simulink model "power_3pfault_parametertest"  (R2017b)
settings: Solver=FixedStepDiscrete  StartTime=0.0  StopTime=0.2  FixedStep=Ts  RelTol=1e-4  EnableMultiTasking=on
PreLoadFcn:
  | Ts=50e-6;
InitFcn:
  | Ts=50e-6;
undefined symbols (not defined in the file or in its folder): D1, Delta
libraries: powerlib x23
Description:
  | Copyright 2008-2017 The MathWorks, Inc.
settings Model: ExtModeTrigMode=oneshot  ExtModeArmWhenConnect=off  ExtModeAutoUpdateStatusClock=off  Creator=MathWorks  LastModifiedBy=estheim
settings DataIOCC: SaveFormat=Array  SignalLoggingSaveFormat=ModelDataLogs  SignalLoggingName=sigsOut
settings OptimizationCC: BlockReduction=off  BooleanDataType=off  ExpressionDepthLimit=2147483647  InitFltsAndDblsToZero=on  EfficientMapNaN2IntZero=off  LifeSpan=inf
settings DebuggingCC: UnderspecifiedInitializationDetection=Classic  MergeDetectMultiDrivingBlocksExec=none  CheckExecutionContextPreStartOutputMsg=on  CheckExecutionContextRuntimeOutputMsg=on  SignalResolutionControl=TryResolveAllWithWarning  MultiTaskDSMMsg=warning  MultiTaskCondExecSysMsg=none  FcnCallInpInsideContextMsg=warning  UnconnectedInputMsg=none  UnconnectedOutputMsg=none  StateNameClashWarn=warning  SFUnexpectedBacktrackingDiag=warning  SFNoUnconditionalDefaultTransitionDiag=warning  SFExecutionAtInitializationDiag=none
settings HardwareCC: ProdBitPerPointer=32  ProdBitPerSizeT=32  ProdBitPerPtrDiffT=32  ProdLargestAtomicFloat=None  ProdIntDivRoundTo=Undefined  ProdEndianess=Unspecified  ProdWordSize=32  ProdHWDeviceType=Specified  TargetUnknown=on
settings ModelReferenceCC: PropagateSignalLabelsOutOfModel=off
settings CodeAppCC: StateflowObjectComments=on
settings GRTTargetCC: TargetLangStandard=C89/C90 (ANSI)  GeneratePreprocessorConditionals=Disable all  CombineOutputUpdateFcns=off  GRTInterface=on
settings ConfigComp: CovMetricSettings=dw  CovHtmlReporting=on  CovSaveCumulativeToWorkspaceVar=on  CovSaveSingleToWorkspaceVar=on  CovExternalEMLEnable=off  CovSFcnEnable=off
settings SimscapeCC: SimscapeNormalizeSystem=off

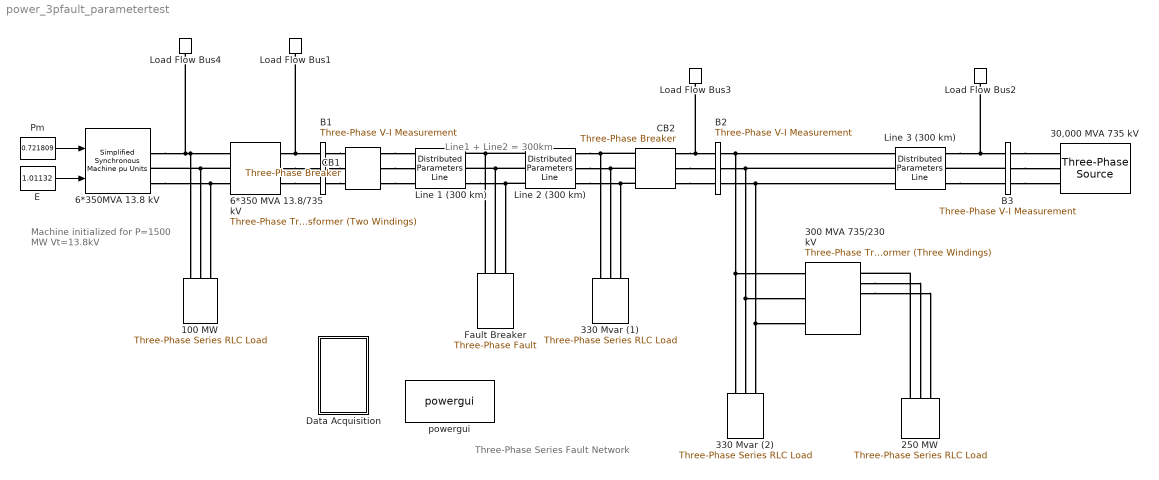
== system power_3pfault_parametertest ==
  note: Line1 + Line2 = 300km
  note: Machine initialized for
      |  P=1500 MW
      |  Vt=13.8kV
  note: Three-Phase Series Fault Network
  100 MW : powerlib/Elements/Three-Phase Series RLC Load  LConnTagsString=A|B|C  Configuration=Y (grounded)  NominalVoltage=13.8e3  Vabc=[1e3 1e3 1e3]  Vabcp=[1e3 1e3 1e3]  NominalFrequency=60  UnbalancedPower=off  ActivePower=100000000  InductivePower=0  CapacitivePower=0  Pabc=[10e3 9e3 11e3]  QLabc=[100 90 110]  QCabc=[100 90 110]  Pabcp=[10e3 9e3 11e3]  QLabcp=[100 90 110]  QCabcp=[100 90 110]  Measurements=None  LoadType=constant Z
  250 MW : powerlib/Elements/Three-Phase Series RLC Load  LConnTagsString=A|B|C  Configuration=Y (grounded)  NominalVoltage=230e3  Vabc=[1e3 1e3 1e3]  Vabcp=[1e3 1e3 1e3]  NominalFrequency=60  UnbalancedPower=off  ActivePower=250000000  InductivePower=0  CapacitivePower=0  Pabc=[10e3 9e3 11e3]  QLabc=[100 90 110]  QCabc=[100 90 110]  Pabcp=[10e3 9e3 11e3]  QLabcp=[100 90 110]  QCabcp=[100 90 110]  Measurements=None  LoadType=constant Z
  30,000 MVA 735 kV : powerlib/Electrical Sources/Three-Phase Source  InternalConnection=Yg  VoltagePhases=off  Voltage=(735000)*0.98865  PhaseAngle=-2.0892  Voltage_phases=[25e3 25e3 25e3]/sqrt(3)  PhaseAngles_phases=[0 -120 +120]  Frequency=60  NonIdealSource=on  SpecifyImpedance=on  Resistance=735^2/30000/10  Inductance=735^2/30000/377  ShortCircuitLevel=30000e6  BaseVoltage=735e3  XRratio=10  BusType=swing  Pref=0  Qref=0  Prefabc=[10e3, 10e3, 10e3]  Qrefabc=[0, 0, 0]  Qmin=-Inf  Qmax=Inf
  300 MVA 735/230 kV : powerlib/Elements/Three-Phase Transformer (Three Windings)  Winding1Connection=Yg  Winding2Connection=Yg  Winding3Connection=Delta (D1)  CoreType=Three single-phase transformers  SetSaturation=on  Hysteresis=off  DataFile='hysteresis'  SetInitialFlux=off  Measurements=None  UNITS=pu  NominalPower=[ 300e6 , 60 ]  Winding1=[ 735e3 , 0.002 , 0.15 ]  Winding2=[ 230e3 , 0.002 , 0 ]  Winding3=[ 25e3 , 0.05 , 0.20 ]  Rm=500  Lm=1000  L0=0.5  Saturation="[  0,0  ;  0.0012,1.2  ;  1.0,1.45 ]"  InitialFluxes=[-1.0077512712612 0.407399313381507 0.600351957879682]  MoreParameters=on  BreakLoop=on  DataType=off  TransfoNumber=0
      settings: AttributesFormatString=\n  SourceProductName=Simscape Power Systems  SourceProductBaseCode=PS
  330 Mvar (1) : powerlib/Elements/Three-Phase Series RLC Load  LConnTagsString=A|B|C  Configuration=Y (grounded)  NominalVoltage=735e3  Vabc=[1e3 1e3 1e3]  Vabcp=[1e3 1e3 1e3]  NominalFrequency=60  UnbalancedPower=off  ActivePower=1320000  InductivePower=330e6  CapacitivePower=0  Pabc=[10e3 9e3 11e3]  QLabc=[100 90 110]  QCabc=[100 90 110]  Pabcp=[10e3 9e3 11e3]  QLabcp=[100 90 110]  QCabcp=[100 90 110]  Measurements=None  LoadType=constant Z
  "330 Mvar (2) " : powerlib/Elements/Three-Phase Series RLC Load  LConnTagsString=A|B|C  Configuration=Y (grounded)  NominalVoltage=735e3  Vabc=[1e3 1e3 1e3]  Vabcp=[1e3 1e3 1e3]  NominalFrequency=60  UnbalancedPower=off  ActivePower=1320000  InductivePower=330e6  CapacitivePower=0  Pabc=[10e3 9e3 11e3]  QLabc=[100 90 110]  QCabc=[100 90 110]  Pabcp=[10e3 9e3 11e3]  QLabcp=[100 90 110]  QCabcp=[100 90 110]  Measurements=None  LoadType=constant Z
  6*350 MVA 13.8/735 kV : powerlib/Elements/Three-Phase Transformer (Two Windings)  Winding1Connection=Delta (D1)  Winding2Connection=Yg  CoreType=Three single-phase transformers  SetSaturation=off  Hysteresis=off  DataFile='hysteresis'  SetInitialFlux=off  Measurements=None  UNITS=pu  NominalPower=[ 6*350e6 , 60 ]  Winding1=[ 13.8e3 , 0.002 , 0.08 ]  Winding2=[ 735e3 , 0.002 , 0.08 ]  Rm=500  Lm=500  L0=0.5  Saturation=[ 0,0 ; 0.0024,1.2 ; 1.0,1.52 ]  InitialFluxes=[ 0.8 , -0.8 , 0.7 ]  MoreParameters=off  BreakLoop=off  DataType=off  TransfoNumber=0
  6*350MVA 13.8 kV : powerlib/Machines/Simplified Synchronous Machine pu Units  ConnectionType=3-wire Y  MechanicalLoad=Mechanical power Pm  MeasurementBus=off  NominalParameters="[ 6*350e6 13.8e3  60 ]"  Mechanical=[ inf,0,2 ]  InternalRL="[ 0.22/15  0.22 ]"  InitialConditions=[0 1.43122 0.716215 0.716215 0.716215 -3.34575 -123.346 116.654 ]  Units=0  LoadFlowParameters=[1,0,0,0,0]  TsPowergui=0  TsBlock=-1  BusType=PV  Pref=1500000000  Qref=0  Qmin=-Inf  Qmax=Inf  PLF=0  QLF=0
      settings: AttributesFormatString=\n  SourceProductName=Simscape Power Systems  SourceProductBaseCode=PS
  B1 : powerlib/Measurements/Three-Phase V-I Measurement  VoltageMeasurement=phase-to-ground  SetLabelV=on  LabelV=Vabc_B1  Vpu=on  VpuLL=off  CurrentMeasurement=yes  SetLabelI=on  LabelI=Iabc_B1  Ipu=on  Pbase=100e6  Vbase=735e3  OutputType=Complex  PhasorSimulation=off  PSBequivalent=0
  B2 : powerlib/Measurements/Three-Phase V-I Measurement  VoltageMeasurement=phase-to-ground  SetLabelV=on  LabelV=Vabc_B2  Vpu=on  VpuLL=off  CurrentMeasurement=yes  SetLabelI=on  LabelI=Iabc_B2  Ipu=on  Pbase=100e6  Vbase=735e3  OutputType=Complex  PhasorSimulation=off  PSBequivalent=0
  B3 : powerlib/Measurements/Three-Phase V-I Measurement  VoltageMeasurement=no  SetLabelV=on  LabelV=Vabc_B3  Vpu=on  VpuLL=off  CurrentMeasurement=no  SetLabelI=on  LabelI=Iabc_B3  Ipu=on  Pbase=100e6  Vbase=735e3  OutputType=Complex  PhasorSimulation=off  PSBequivalent=0
  CB1 : powerlib/Elements/Three-Phase Breaker  InitialState=closed  SwitchA=on  SwitchB=on  SwitchC=on  SwitchTimes="[5/60  ]"  External=off  BreakerResistance=0.001  SnubberResistance=1e5  SnubberCapacitance=inf  Measurements=None
      settings: AttributesFormatString=\n
  CB2 : powerlib/Elements/Three-Phase Breaker  InitialState=closed  SwitchA=on  SwitchB=on  SwitchC=on  SwitchTimes="[5/60  ]"  External=off  BreakerResistance=0.001  SnubberResistance=1e5  SnubberCapacitance=inf  Measurements=None
      settings: AttributesFormatString=\n
  Data Acquisition : Subsystem  mask(Data Acquisition){}
      mask Display: disp('Scopes')
  E : Constant  Value=1.01132
  Fault Breaker : powerlib/Elements/Three-Phase Fault  InitialStates=0  FaultA=off  FaultB=on  FaultC=off  GroundFault=on  SwitchTimes=faultinception2  External=off  SwitchStatus=NaN  FaultResistance=faultres  GroundResistance=1  SnubberResistance=inf  SnubberCapacitance=inf  Measurements=Fault voltages and currents
  Line 1 (300 km) : powerlib/Elements/Distributed Parameters Line  Phases=3  Frequency=60  Resistance=[0.01273 0.3864]  Inductance="[0.9337e-3  4.1264e-3]"  Capacitance=[12.74e-9 7.751e-9]  Length=line1  x1=[-0.0003 -3.78759842950766e-08 628975.403312343 -495883.769880965;-0.00025 -3.75285463548764e-08 638210.318952053 -483940.521945147;-0.0002 -3.71677747008528e-08 647218.481504353 -471825.332246222;-0.00015 -3.67937975134568e-08 655996.690411981 -459542.505253402;-0.0001 -3.64067476650022e-08 664541.826819112 -447096.404996632;-5e-05 -3.60067626724573e-08 672850.854679469 -434491.453516068]  x2=[-0.0003 -3.45807686958301e-08 605295.232742086 -519409.81725687;-0.00025 -3.4265507824739e-08 614977.783461343 -507908.720868203;-0.0002 -3.39380725818771e-08 624441.835502426 -496227.166929478;-0.00015 -3.3598579303427e-08 633684.026332709 -484369.305841187;-0.0001 -3.32471486097339e-08 642701.072245797 -472339.350644913;-5e-05 -3.28839053624501e-08 651489.769528212 -460141.575526454]  x3=[-0.0003 -2.61251237348243e-11 876.888880838957 -609.09527519692;-0.00025 -2.50551766038549e-11 888.21347189918 -592.459310580762;-0.0002 -2.39763274879413e-11 899.22248494217 -575.612847992619;-0.00015 -2.28889596970374e-11 909.912008518013 -558.561872900433;-0.0001 -2.17934595677416e-11 920.278244689884 -541.312443434463;-5e-05 -2.06902163260335e-11 930.31751038343 -523.870688234865]  x4=[-0.0003 -7.92696517991683e-11 3552.49798963012 -3282.73159030779;-0.00025 -7.95960668313405e-11 3613.74152071813 -3215.18949934517;-0.0002 -7.98942017599735e-11 3673.7011066511 -3146.50506686293;-0.00015 -8.0163950659147e-11 3732.35544407363 -3076.70269611289;-0.0001 -8.04052176883613e-11 3789.68369337894 -3005.80718754501;-5e-05 -8.06179171265899e-11 3845.66548611301 -2933.8437299959]  x5=0.000282770783497871  V1=ones(3,3)  V2=ones(3,3)  I1=ones(3,3)  I2=ones(3,3)  nHarmo=1  Measurements=None
      settings: AttributesFormatString=\n  SourceProductName=Simscape Power Systems
  Line 2 (300 km) : powerlib/Elements/Distributed Parameters Line  Phases=3  Frequency=60  Resistance=[0.01273 0.3864]  Inductance="[0.9337e-3  4.1264e-3]"  Capacitance=[12.74e-9 7.751e-9]  Length=line2  x1=[-0.00145 -3.82709877736309e-08 0 0;-0.0014 -3.82574787054797e-08 0 0;-0.00135 -3.8230376937312e-08 0 0;-0.0013 -3.81896920982569e-08 0 0;-0.00125 -3.8135438643444e-08 0 0;-0.0012 -3.80676358488675e-08 0 0;-0.00115 -3.79863078045374e-08 0 0;-0.0011 -3.78914834059206e-08 0 0;-0.00105 -3.77831963436745e-08 0 0;-0.001 -3.76614850916767e-08 0 0;-0.00095 -3.75263928933554e-08 0 0;-0.0009 -3.73779677463254e-08 473387.852694452 -641928.29724098;-0.00085 -3.72162623853347e-08 485403.128607504 -632891.679417048;-0.0008 -3.70413342635282e-08 497245.943100267 -623630.198193008;-0.00075 -3.68532455320345e-08 508912.088477141 -614147.144129039;-0.0007 -3.66520630178844e-08 520397.419812224 -604445.886509095;-0.00065 -3.64378582002671e-08 531697.856421981 -594529.872143814;-0.0006 -3.62107071851344e-08 542809.383315095 -584402.624145885;-0.00055 -3.59706906781605e-08 553728.052618967 -574067.740678299;-0.0005 -3.57178939560672e-08 564449.984982385 -563528.893675942;-0.00045 -3.54524068363264e-08 574971.370953834 -552789.82754097;-0.0004 -3.51743236452474e-08 585288.472334977 -541854.357812448;-0.00035 -3.48837431844639e-08 595397.62350882 -530726.369810698;-0.0003 -3.45807686958301e-08 605295.232742086 -519409.81725687;-0.00025 -3.4265507824739e-08 614977.783461343 -507908.720868203;-0.0002 -3.39380725818771e-08 624441.835502426 -496227.166929478;-0.00015 -3.3598579303427e-08 633684.026332709 -484369.305841187;-0.0001 -3.32471486097339e-08 642701.072245797 -472339.350644913;-5e-05 -3.28839053624501e-08 651489.769528212 -460141.575526454]  x2=[-0.00145 -1.47649338361576e-08 0 0;-0.0014 -1.47608425428165e-08 0 0;-0.00135 -1.47515067924054e-08 0 0;-0.0013 -1.4736929901872e-08 0 0;-0.00125 -1.47171170503161e-08 0 0;-0.0012 -1.46920752771496e-08 0 0;-0.00115 -1.46618134795951e-08 0 0;-0.0011 -1.46263424095253e-08 0 0;-0.00105 -1.45856746696424e-08 0 0;-0.001 -1.45398247090008e-08 0 0;-0.00095 -1.44888088178732e-08 0 0;-0.0009 -1.44326451219628e-08 305808.693622115 -687287.971048075;-0.00085 -1.43713535759632e-08 318708.688794987 -681401.883166662;-0.0008 -1.43049559564691e-08 331495.448288299 -675273.696440736;-0.00075 -1.42334758542383e-08 344164.429027289 -668905.58818586;-0.0007 -1.41569386658109e-08 356711.129783425 -662299.820960574;-0.00065 -1.40753715844855e-08 369131.092773671 -655458.74176252;-0.0006 -1.39888035906577e-08 381419.905244316 -648384.781194561;-0.00055 -1.38972654415234e-08 393573.201038804 -641080.452601205;-0.0005 -1.38007896601512e-08 405586.662149007 -633548.35117562;-0.00045 -1.36994105239269e-08 417456.020249398 -625791.153037578;-0.0004 -1.35931640523748e-08 429177.058213561 -617811.614282639;-0.00035 -1.34820879943603e-08 440745.611612517 -609612.570002929;-0.0003 -1.3366221814678e-08 452157.57019433 -601196.933279839;-0.00025 -1.32456066800298e-08 463408.879344454 -592567.694149025;-0.0002 -1.31202854443986e-08 474495.541526323 -583727.918538061;-0.00015 -1.29903026338229e-08 485413.617701655 -574680.747177129;-0.0001 -1.28557044305762e-08 496159.228729971 -565429.394483136;-5e-05 -1.27165386567593e-08 506728.55674684 -555977.147417641]  x3=[-0.00145 -3.38199281059364e-11 0 0;-0.0014 -3.30171295486336e-11 0 0;-0.00135 -3.22026001624171e-11 0 0;-0.0013 -3.13766293456994e-11 0 0;-0.00125 -3.05395105619787e-11 0 0;-0.0012 -2.96915412355729e-11 0 0;-0.00115 -2.88330226459457e-11 0 0;-0.0011 -2.79642598206644e-11 0 0;-0.00105 -2.70855614270239e-11 0 0;-0.001 -2.61972396623794e-11 0 0;-0.00095 -2.52996101432242e-11 0 0;-0.0009 -2.43929917930521e-11 757.656727728583 -729.222631766939;-0.00085 -2.34777067290461e-11 771.266751177753 -714.812683047661;-0.0008 -2.25540801476311e-11 784.602747222709 -700.148764785762;-0.00075 -2.16224402089336e-11 797.659977647554 -685.236087001576;-0.0007 -2.06831179201877e-11 810.433803280494 -670.07994809851;-0.00065 -1.97364470181298e-11 822.919685642104 -654.68573298055;-0.0006 -1.87827638504238e-11 835.113188557834 -639.058911139025;-0.00055 -1.78224072561581e-11 847.00997973416 -623.205034709326;-0.0005 -1.68557184454577e-11 858.605832297825 -607.12973649826;-0.00045 -1.58830408782542e-11 869.896626297627 -590.838727982736;-0.0004 -1.49047201422556e-11 880.878350168221 -574.337797280508;-0.00035 -1.39211038301611e-11 891.547102155406 -557.632807093684;-0.0003 -1.29325414161627e-11 901.899091702403 -540.729692625733;-0.00025 -1.19393841317789e-11 911.930640796616 -523.634459472741;-0.0002 -1.0941984841064e-11 921.63818527642 -506.353181489645;-0.00015 -9.94069791523649e-12 931.018276097484 -488.891998632227;-0.0001 -8.93587910677354e-12 940.067580558204 -471.257114775611;-5e-05 -7.92788542301321e-12 948.782883483794 -453.454795510062]  x4=[-0.00145 -3.20986509931294e-11 0 0;-0.0014 -3.32576226301539e-11 0 0;-0.00135 -3.4404777992218e-11 0 0;-0.0013 -3.55397095004839e-11 0 0;-0.00125 -3.66620139191907e-11 0 0;-0.0012 -3.77712924989226e-11 0 0;-0.00115 -3.88671511182821e-11 0 0;-0.0011 -3.99492004239198e-11 0 0;-0.00105 -4.10170559688696e-11 0 0;-0.001 -4.20703383491414e-11 0 0;-0.00095 -4.31086733385205e-11 0 0;-0.0009 -4.41316920215295e-11 1294.72060349585 -4606.45046471645;-0.00085 -4.51390309245015e-11 1381.31528161887 -4581.22864876283;-0.0008 -4.61303321447208e-11 1467.41918499962 -4554.37914408437;-0.00075 -4.71052434775842e-11 1553.00172133124 -4525.91149018223;-0.0007 -4.80634185417371e-11 1638.03248354606 -4495.8358014783;-0.00065 -4.90045169021418e-11 1722.48126061917 -4464.16276372154;-0.0006 -4.9928204191032e-11 1806.31804830218 -4430.90363019148;-0.00055 -5.08341522267121e-11 1889.51305978362 -4396.07021769988;-0.0005 -5.17220391301589e-11 1972.03673627207 -4359.67490239234;-0.00045 -5.25915494393834e-11 2053.85975749819 -4321.73061535108;-0.0004 -5.34423742215129e-11 2134.95305213218 -4282.25083800063;-0.00035 -5.42742111825536e-11 2215.28780811258 -4241.24959731787;-0.0003 -5.50867647747943e-11 2294.8354828831 -4198.74146084839;-0.00025 -5.58797463018126e-11 2373.56781353369 -4154.74153153068;-0.0002 -5.66528740210479e-11 2451.45682684215 -4109.26544233011;-0.00015 -5.74058732439029e-11 2528.47484921294 -4062.32935068463;-0.0001 -5.81384764333391e-11 2604.59451650943 -4013.94993276412;-5e-05 -5.88504232989318e-11 2679.78878377629 -3964.14437754538]  x5=0.00141385391748936  V1=ones(3,3)  V2=ones(3,3)  I1=ones(3,3)  I2=ones(3,3)  nHarmo=1  Measurements=None
      settings: AttributesFormatString=\n  SourceProductName=Simscape Power Systems
  Line 3 (300 km) : powerlib/Elements/Distributed Parameters Line  Phases=3  Frequency=60  Resistance=[0.01273 0.3864]  Inductance="[0.9337e-3  4.1264e-3]"  Capacitance=[12.74e-9 7.751e-9]  Length=300  x1=[-0.0017 -1.45723124159187e-08 0 0;-0.00165 -1.45905087920394e-08 0 0;-0.0016 -1.46035212298608e-08 0 0;-0.00155 -1.46113451061256e-08 0 0;-0.0015 -1.46139776410478e-08 0 0;-0.00145 -1.46114178993003e-08 0 0;-0.0014 -1.46036667903472e-08 0 0;-0.00135 -1.45907270681206e-08 0 0;-0.0013 -1.45726033300422e-08 0 0;-0.00125 -1.45493020153897e-08 0 0;-0.0012 -1.45208314030094e-08 0 0;-0.00115 -1.44872016083743e-08 0 0;-0.0011 -1.44484245799902e-08 0 0;-0.00105 -1.44045140951508e-08 266474.832453814 -703471.218755304;-0.001 -1.43554857550421e-08 279686.845489083 -698323.636957029;-0.00095 -1.43013569792e-08 292799.487119911 -692927.944095694;-0.0009 -1.42421469993208e-08 305808.098487165 -687286.057235279;-0.00085 -1.41778768524284e-08 318708.057693168 -681399.980911323;-0.0008 -1.41085693733999e-08 331494.781443838 -675271.806418715;-0.00075 -1.40342491868527e-08 344163.726677113 -668903.711068673;-0.0007 -1.39549426983952e-08 356710.392177076 -662297.957415152;-0.00065 -1.3870678085245e-08 369130.320173217 -655456.892450971;-0.0006 -1.3781485286218e-08 381419.097924258 -648382.946773938;-0.00055 -1.3687395991091e-08 393572.359285978 -641078.633723268;-0.0005 -1.35884436293425e-08 405585.786262486 -633546.548486608;-0.00045 -1.34846633582754e-08 417455.110540379 -625789.367177978;-0.0004 -1.3376092050526e-08 429176.115005258 -617809.845886958;-0.00035 -1.32627682809629e-08 440744.635240049 -609610.81969947;-0.0003 -1.31447323129818e-08 452156.561004597 -601195.201690476;-0.00025 -1.30220260842001e-08 463407.837696017 -592565.981888984;-0.0002 -1.28946931915566e-08 474494.467789275 -583726.226215699;-0.00015 -1.27627788758217e-08 485412.512257488 -574679.075393721;-0.0001 -1.26263300055237e-08 496158.091971445 -565427.743832659;-5e-05 -1.24853950602965e-08 506727.38907784 -555975.518486563]  x2=[-0.0017 -6.87576100037701e-10 0 0;-0.00165 -6.8480237107496e-10 0 0;-0.0016 -6.81785335090544e-10 0 0;-0.00155 -6.78526064022971e-10 0 0;-0.0015 -6.75025715875733e-10 0 0;-0.00145 -6.71285534305859e-10 0 0;-0.0014 -6.67306848182051e-10 0 0;-0.00135 -6.63091071112545e-10 0 0;-0.0013 -6.58639700942858e-10 0 0;-0.00125 -6.53954319223618e-10 0 0;-0.0012 -6.49036590648638e-10 0 0;-0.00115 -6.43888262463464e-10 0 0;-0.0011 -6.38511163844588e-10 0 0;-0.00105 -6.32907205249543e-10 96634.7706415658 -730540.857796646;-0.001 -6.27078377738136e-10 110387.161752313 -728589.667633419;-0.00095 -6.21026752265026e-10 124100.332830112 -726379.613030548;-0.0009 -6.14754478943929e-10 137769.411650574 -723911.479209909;-0.00085 -6.08263786283689e-10 151389.541655082 -721186.143087697;-0.0008 -6.01556980396502e-10 164955.883676299 -718204.572962859;-0.00075 -5.94636444178565e-10 178463.617657503 -714967.828173063;-0.0007 -5.87504636463443e-10 191907.944365128 -711477.05871832;-0.00065 -5.80164091148457e-10 205284.087093914 -707733.504852397;-0.0006 -5.72617416294407e-10 218587.293364039 -703738.496642157;-0.00055 -5.64867293198933e-10 231812.836609661 -699493.453494994;-0.0005 -5.56916475443867e-10 244956.017858239 -694999.883654524;-0.00045 -5.487677879169e-10 258012.16740006 -690259.383664716;-0.0004 -5.40424125807908e-10 270976.646447359 -685273.637802643;-0.00035 -5.3188845358031e-10 283844.848782462 -680044.417480071;-0.0003 -5.23163803917805e-10 296612.202394354 -674573.580614079;-0.00025 -5.14253276646874e-10 309274.171103089 -668863.070966957;-0.0002 -5.05160037635428e-10 321826.256171477 -662914.917455591;-0.00015 -4.95887317667989e-10 334263.99790346 -656731.233430601;-0.0001 -4.86438411297809e-10 346582.977228626 -650314.215925476;-5e-05 -4.76816675676328e-10 358778.817272279 -643666.14487598]  x3=[-0.0017 -1.26865525293809e-11 0 0;-0.00165 -1.22949508567725e-11 0 0;-0.0016 -1.18989808466686e-11 0 0;-0.00155 -1.14987831853282e-11 0 0;-0.0015 -1.10945000610749e-11 0 0;-0.00145 -1.06862751137777e-11 0 0;-0.0014 -1.02742533838165e-11 0 0;-0.00135 -9.85858126055014e-12 0 0;-0.0013 -9.43940643030468e-12 0 0;-0.00125 -9.01687782390138e-12 0 0;-0.0012 -8.59114556374218e-12 0 0;-0.00115 -8.16236091047193e-12 0 0;-0.0011 -7.73067620923624e-12 0 0;-0.00105 -7.29624483555393e-12 146.058519777444 -1136.85216743786;-0.001 -6.85922114082348e-12 167.460346140684 -1133.89743393128;-0.00095 -6.41976039748269e-12 188.802674640324 -1130.53983206561;-0.0009 -5.97801874384112e-12 210.077922448669 -1126.7805547808;-0.00085 -5.5341531286049e-12 231.27853057148 -1122.62093773017;-0.0008 -5.08832125511361e-12 252.396966533639 -1118.06245880587;-0.00075 -4.64068152530903e-12 273.425727055406 -1113.10673761373;-0.0007 -4.19139298345565e-12 294.357340718299 -1107.75553489791;-0.00065 -3.74061525963306e-12 315.184370619652 -1102.01075191526;-0.0006 -3.28850851302011e-12 335.899417014911 -1095.87442975979;-0.00055 -2.83523337499111e-12 356.49511994673 -1089.34874863758;-0.0005 -2.38095089204426e-12 376.964161859926 -1082.43602709203;-0.00045 -1.92582246858266e-12 397.299270201372 -1075.1387211802;-0.0004 -1.47000980956799e-12 417.493220003902 -1067.45942360014;-0.00035 -1.01367486306761e-12 437.538836453309 -1059.40086276971;-0.0003 -5.56979762715121e-13 457.428997437517 -1050.9659018572;-0.00025 -1.0008677010506e-13 477.156636077037 -1042.15753776405;-0.0002 3.56841782857845e-13 496.714743235796 -1032.9789000601;-0.00015 8.13643551634444e-13 516.09637001145 -1023.4332498716;-0.0001 1.27015623673141e-12 535.294630204293 -1013.52397872262;-5e-05 1.72621764136546e-12 554.302702763892 -1003.25460733002]  x4=[-0.0017 -4.82541696893376e-12 0 0;-0.00165 -5.35583900695815e-12 0 0;-0.0016 -5.88435814088582e-12 0 0;-0.00155 -6.41078659038511e-12 0 0;-0.0015 -6.93493731793454e-12 0 0;-0.00145 -7.45662409527644e-12 0 0;-0.0014 -7.97566156958288e-12 0 0;-0.00135 -8.49186532931071e-12 0 0;-0.0013 -9.00505196972204e-12 0 0;-0.00125 -9.51503915804716e-12 0 0;-0.0012 -1.00216456982664e-11 0 0;-0.00115 -1.05246915954883e-11 0 0;-0.0011 -1.10239981199009e-11 0 0;-0.00105 -1.15193878702735e-11 141.875750296584 -4366.85509796771;-0.001 -1.20106848369868e-11 224.159158139472 -4363.40508133909;-0.00095 -1.24977144645678e-11 306.362923300832 -4358.40476766195;-0.0009 -1.29803037137088e-11 388.457839174327 -4351.85593352391;-0.00085 -1.34582811227476e-11 470.414737827251 -4343.76090569457;-0.0008 -1.39314768685867e-11 552.204500363761 -4334.12256029876;-0.00075 -1.43997228270308e-11 633.798067270678 -4322.94432179472;-0.0007 -1.48628526325204e-11 715.166448742199 -4310.23016175735;-0.00065 -1.53207017372409e-11 796.28073497983 -4295.98459746718;-0.0006 -1.57731074695855e-11 877.112106463908 -4280.21269030536;-0.00055 -1.62199090919516e-11 957.631844193032 -4262.92004395542;-0.0005 -1.66609478578504e-11 1037.81133988779 -4244.11280241226;-0.00045 -1.70960670683084e-11 1117.62210615515 -4223.79764779925;-0.0004 -1.7525112127542e-11 1197.03578660988 -4201.98179799408;-0.00035 -1.79479305978845e-11 1276.02416594946 -4178.67300406432;-0.0003 -1.83643722539467e-11 1354.55917997881 -4153.87954751346;-0.00025 -1.87742891359913e-11 1432.61292558141 -4127.61023733856;-0.0002 -1.91775356025019e-11 1510.15767063311 -4099.87440690043;-0.00015 -1.95739683819289e-11 1587.16586385522 -4070.68191060756;-0.0001 -1.99634466235937e-11 1663.61014460339 -4040.04312041489;-5e-05 -2.03458319477314e-11 1739.46335258865 -4007.96892213868]  x5=0.00169662470098723  V1=ones(3,3)  V2=ones(3,3)  I1=ones(3,3)  I2=ones(3,3)  nHarmo=1  Measurements=None
      settings: AttributesFormatString=\n  SourceProductName=Simscape Power Systems
  Load Flow Bus1 : powerlib/Measurements/Load Flow Bus  LConnTagsString=a  Phases=single  Connectors=on one side  ID=B1  Vbase=735e3  Vref=1  Vangle=0  VLF=1.012  VLFb=1  VLFc=1  angleLF=16.39  angleLFb=0  angleLFc=0
      settings: AttributesFormatString=%<ID>\n%<Vbase>V\n%<VLF>pu\n%<angleLF>deg.  SourceProductName=Simscape Power Systems
  Load Flow Bus2 : powerlib/Measurements/Load Flow Bus  LConnTagsString=a  Phases=single  Connectors=on one side  ID=B3  Vbase=735e3  Vref=1  Vangle=0  VLF=1  VLFb=1  VLFc=1  angleLF=0  angleLFb=0  angleLFc=0
      settings: AttributesFormatString=%<ID>\n%<Vbase>V\n%<VLF>pu\n%<angleLF>deg.  SourceProductName=Simscape Power Systems
  Load Flow Bus3 : powerlib/Measurements/Load Flow Bus  LConnTagsString=a  Phases=single  Connectors=on one side  ID=B2  Vbase=735e3  Vref=1  Vangle=0  VLF=1.03  VLFb=1  VLFc=1  angleLF=7.354  angleLFb=0  angleLFc=0
      settings: AttributesFormatString=%<ID>\n%<Vbase>V\n%<VLF>pu\n%<angleLF>deg.  SourceProductName=Simscape Power Systems
  Load Flow Bus4 : powerlib/Measurements/Load Flow Bus  LConnTagsString=a  Phases=single  Connectors=on one side  ID=GEN  Vbase=13.8e3  Vref=1  Vangle=0  VLF=1  VLFb=1  VLFc=1  angleLF=-7.552  angleLFb=0  angleLFc=0
      settings: AttributesFormatString=%<ID>\n%<Vbase>V\n%<VLF>pu\n%<angleLF>deg.  SourceProductName=Simscape Power Systems
  Pm : Constant  Value=0.721809
  powergui : powerlib/powergui  Priority=2  SimulationMode=Discrete  SampleTime=Ts  frequency=60  Iterations=50  frequencyindice=60  Pbase=100e6  ErrMax=0.0001  UnitsV=kV  UnitsW=MW  buscounter=0  FunctionMessages=off  echomessages=off  EnableUseOfTLC=off  CurrentSourceSwitches=off  DisableSnubberDevices=off  DisableRonSwitches=off  DisableVfSwitches=off  DisplayEquations=off  SolverType=Tustin/Backward Euler (TBE)  Interpol=off  ExternalGateDelay=off  methode=off  Ts=0  x0status=blocks  SPID=off  SwTol=0  HookPort=off  RestoreLinks=warning  ResistiveCurrentMeasurement=off  Frange=0:0.5:500  Ylog=off  Xlog=off  ShowGrid=off  save=on  variable=Zmes  structure=0  ZoomFFT=on  StartTime=0.0  cycles=1  DisplayStyle=off  fundamental=60  FreqAxis=off  MaxFrequency=1000  frequencyindicesteady=1  RmsSteady=1  display=off
  wires:
  Pm/1 -> 6*350MVA 13.8 kV/1
  E/1 -> 6*350MVA 13.8 kV/2
  connections:
  6*350 MVA 13.8/735 kV/LConn2 -- 6*350MVA 13.8 kV/RConn2 -- 100 MW/LConn2
  6*350MVA 13.8 kV/RConn1 -- 6*350 MVA 13.8/735 kV/LConn1 -- 100 MW/LConn1 -- Load Flow Bus4/LConn1
  6*350MVA 13.8 kV/RConn3 -- 6*350 MVA 13.8/735 kV/LConn3 -- 100 MW/LConn3
  6*350 MVA 13.8/735 kV/RConn2 -- B1/LConn2
  6*350 MVA 13.8/735 kV/RConn1 -- B1/LConn1 -- Load Flow Bus1/LConn1
  6*350 MVA 13.8/735 kV/RConn3 -- B1/LConn3
  B1/RConn2 -- CB1/LConn2
  B1/RConn1 -- CB1/LConn1
  B1/RConn3 -- CB1/LConn3
  CB1/RConn2 -- Line 1 (300 km)/LConn2
  CB1/RConn1 -- Line 1 (300 km)/LConn1
  CB1/RConn3 -- Line 1 (300 km)/LConn3
  CB2/LConn1 -- Line 2 (300 km)/RConn1 -- 330 Mvar (1)/LConn1
  Line 1 (300 km)/RConn3 -- Line 2 (300 km)/LConn3 -- Fault Breaker/LConn3
  CB2/RConn2 -- B2/LConn2
  CB2/RConn1 -- B2/LConn1 -- Load Flow Bus3/LConn1
  CB2/RConn3 -- B2/LConn3
  CB2/LConn2 -- Line 2 (300 km)/RConn2 -- 330 Mvar (1)/LConn2
  B2/RConn2 -- Line 3 (300 km)/LConn2 -- "330 Mvar (2) "/LConn2 -- 300 MVA 735/230 kV/LConn2
  300 MVA 735/230 kV/RConn2 -- 250 MW/LConn2
  250 MW/LConn1 -- 300 MVA 735/230 kV/RConn1
  300 MVA 735/230 kV/RConn3 -- 250 MW/LConn3
  Line 3 (300 km)/RConn1 -- B3/LConn1 -- Load Flow Bus2/LConn1
  B3/LConn2 -- Line 3 (300 km)/RConn2
  Line 3 (300 km)/RConn3 -- B3/LConn3
  B3/RConn3 -- 30,000 MVA 735 kV/RConn3
  B3/RConn2 -- 30,000 MVA 735 kV/RConn2
  B3/RConn1 -- 30,000 MVA 735 kV/RConn1
  B2/RConn1 -- Line 3 (300 km)/LConn1 -- "330 Mvar (2) "/LConn1 -- 300 MVA 735/230 kV/LConn1
  B2/RConn3 -- Line 3 (300 km)/LConn3 -- "330 Mvar (2) "/LConn3 -- 300 MVA 735/230 kV/LConn3
  Fault Breaker/LConn1 -- Line 2 (300 km)/LConn1 -- Line 1 (300 km)/RConn1
  Fault Breaker/LConn2 -- Line 2 (300 km)/LConn2 -- Line 1 (300 km)/RConn2
  CB2/LConn3 -- Line 2 (300 km)/RConn3 -- 330 Mvar (1)/LConn3

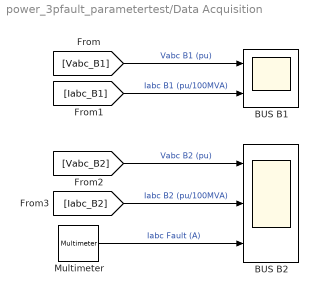
== system power_3pfault_parametertest/Data Acquisition ==
  BUS B1 : Scope  NumInputPorts=2
  BUS B2 : Scope  NumInputPorts=3
  Multimeter : powerlib/Measurements/Multimeter  Tag=PoWeRsYsTeMmEaSuReMeNt  PhasorSimulation=off  OutputType=Magnitude  sel=4  L=6  Gain=1  yselected={'Ib: Fault Breaker/Fault A'};  PSBOutputType=1  PSBequivalent=0  AxesSetting=[0,0.1,-100,100]  Display=0  SavedBlockNames={}
      settings: AttributesFormatString=\n
  wires:
  [Vabc_B1] -> BUS B1/1  "Vabc B1 (pu)"
  [Iabc_B1] -> BUS B1/2  "Iabc B1 (pu/100MVA)"
  [Vabc_B2] -> BUS B2/1  "Vabc B2 (pu)"
  [Iabc_B2] -> BUS B2/2  "Iabc B2 (pu/100MVA)"
  Multimeter/1 -> BUS B2/3  "Iabc Fault (A)"
